simulink model "studycase"  (R2021a)
settings: Solver=VariableStepAuto  StartTime=0.0  StopTime=10.0  RelTol=1e-3
settings Model: Creator=surya  LastModifiedBy=surya

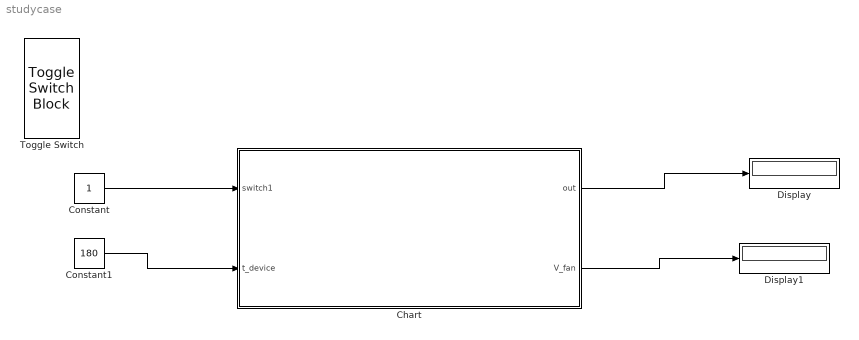
== system studycase ==
  Chart : Stateflow chart  TreatAsAtomicUnit=on
  Constant : Constant
  Constant1 : Constant  Value=180
  Display : Display
  Display1 : Display
  Toggle Switch : ToggleSwitchBlock
      settings: Values={{'Off', 'On'}, [0 1]}
  wires:
  Constant/1 -> Chart/1(switch1)
  Chart/1(out) -> Display/1
  Constant1/1 -> Chart/2(t_device)
  Chart/2(V_fan) -> Display1/1

== stateflow chart studycase/Chart ==
  state SystemStatus [parallel]
    settings: executionOrder=1
    state SystemOff
      en:
      out=0;
    state SystemOn
      en:
      out=1;
      du:FanTable(t_device);
    (default) -> SystemOff
    SystemOff -> SystemOn : [switch1&&iscool(t_device)]
    SystemOn -> SystemOff : [~switch1&&~iscool(t_device)]{fan_mode=Off}
  state FANlogic [parallel]
    settings: executionOrder=2
    state FanOFF
      en:V_fan=0
    state FanOn
      en:V_fan=0.75
    state FanHi
      en:V_fan=1;
    (default) -> FanOFF
    FanOFF -> FanOn [order 1] : [fan_mode==Lo]
    FanOn -> FanOFF [order 1] : [fan_mode==Off]
    FanOn -> FanHi [order 2] : [fan_mode==Hi]
    FanHi -> FanOn [order 1] : [fan_mode==Lo]
    FanOFF -> FanHi [order 2] : [fan_mode==Hi]
    FanHi -> FanOFF [order 2] : [fan_mode==Off]
  state status=iscool(t) [function]
    (default) -> (junction 24)
    (junction 24) -> (junction 25) [order 1] : [t<=160]
    (junction 24) -> (junction 26) [order 2] : {status=0;}
    (junction 25) -> (junction 27) : {status=1;}
    (junction 27) -> (junction 26)
    (junction 26) -> (junction 28)
  data: t function_input; status function_output; T function_input; switch1 input; out output; t_device input; fan_mode local Enum: fan_mode_type; V_fan output
  function FanTable(T):
    | function FanTable(T)
    | 
    | aVarTruthTableCondition_1 = false;
    | aVarTruthTableCondition_2 = false;
    | aVarTruthTableCondition_3 = false;
    | 
    | 
    | % Device is cold
    | 
    | aVarTruthTableCondition_1 = logical(T<50);
    | 
    | % Device is lukewarm
    | 
    | aVarTruthTableCondition_2 = logical(T<120);
    | 
    | % Device is warm
    | 
    | aVarTruthTableCondition_3 = logical(T<160);
    | 
    | if (aVarTruthTableCondition_1)
    |     A1();
    | elseif (aVarTruthTableCondition_2)
    |     A2();
    | elseif (aVarTruthTableCondition_3)
    |     A3();
    | else % Default
    |     A1();
    | end
    | 
    | function A1()
    | 
    | % No Fan
    | 
    | fan_mode=Off;
    | 
    | function A2()
    | 
    | % Low fan
    | 
    | fan_mode=Lo;
    | 
    | function A3()
    | 
    | % High fan
    | 
    | fan_mode=Hi;
